simulink model "dc_motor"  (R2024a)
settings: Solver=ode15s  StartTime=0.0  StopTime=10.0  RelTol=1e-3
model workspace (MAT data in the model file):
  J = 5e-05
  K = 0.2
  L = 0.01
  R = 4
  V = 7.4
  b = 0.0005
settings Model: Creator=Admin  LastModifiedBy=Admin

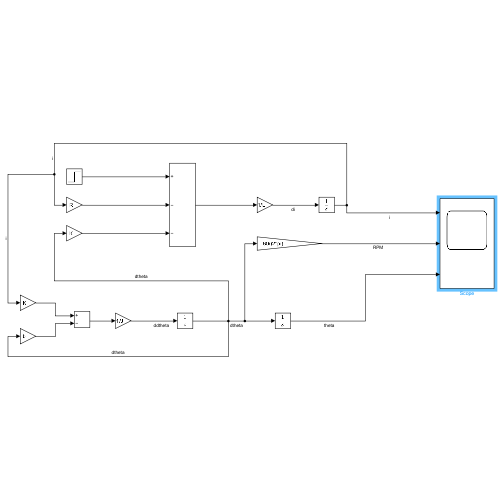
[thumbnail: Simulink's stored preview of the top-level diagram]
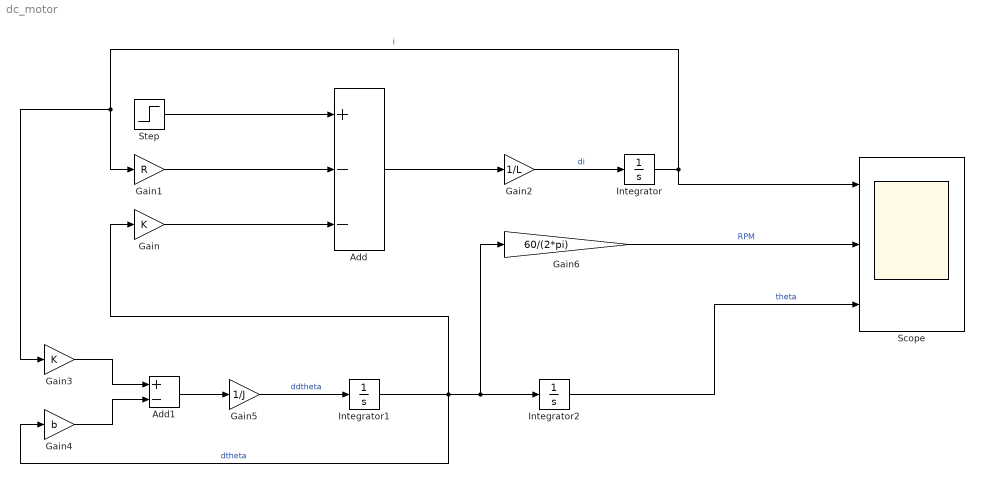
== system dc_motor ==
  Add : Sum  Inputs=+--
  Add1 : Sum  Inputs=+-
  Gain : Gain  Gain=K
  Gain1 : Gain  Gain=R
  Gain2 : Gain  Gain=1/L
  Gain3 : Gain  Gain=K
  Gain4 : Gain  Gain=b
  Gain5 : Gain  Gain=1/J
  Gain6 : Gain  Gain=60/(2*pi)
  Integrator : Integrator
  Integrator1 : Integrator
  Integrator2 : Integrator
  Scope : Scope  NumInputPorts=3
  Step : Step  After=V  SampleTime=0
  wires:
  Integrator/1 -> Gain3/1, Gain1/1, Scope/1  "i"
  Integrator1/1 -> Gain4/1, Integrator2/1, Gain6/1, Gain/1  "dtheta"
  Integrator2/1 -> Scope/3  "theta"
  Gain5/1 -> Integrator1/1  "ddtheta"
  Gain2/1 -> Integrator/1  "di"
  Step/1 -> Add/1
  Gain/1 -> Add/3
  Gain1/1 -> Add/2
  Add/1 -> Gain2/1
  Gain3/1 -> Add1/1
  Gain4/1 -> Add1/2
  Add1/1 -> Gain5/1
  Gain6/1 -> Scope/2  "RPM"
